simulink model "example"  (R2020a)
settings: Solver=VariableStepAuto  StartTime=0.0  StopTime=10.0  RelTol=1e-3
settings Model: Creator=Laura  LastModifiedBy=Laura

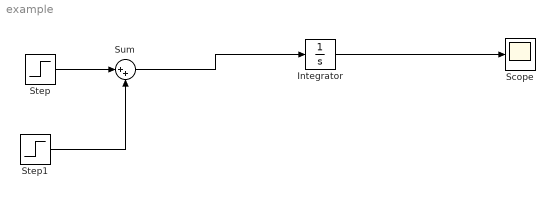
== system example ==
  Integrator : Integrator
  Scope : Scope
  Step : Step  SampleTime=0
  Step1 : Step  Time=2  After=-1  SampleTime=0
  Sum : Sum  Inputs=|++
  wires:
  Step/1 -> Sum/1
  Step1/1 -> Sum/2
  Sum/1 -> Integrator/1
  Integrator/1 -> Scope/1
